simulink model "D_FB_J_controlled"  (R2020b)
(part 4 of 4)

                                                                                                                                                                                                                                                                                                                                                                                                                                                                                                                                                                                                                                                                                                                                                                                                                                                                                                                                                                                                                                                                                                                                                                                                                                                                                                                                                                                                                                                                                                                                                                                                                                                                                                                                                                                                                                                                                                                                                                                                                                                                                                                                                                                                  0.5000*a3B*dalfa*ml3B*offB*sin(th1B + th2B + th3B) + 0.5000*a3B*dbeta*ml3B*offB*sin(th1B + th2B + th3B) + 0.5000*L*a3B*dalfa*ml3B*sin(beta + th1B + th2B + th3B) + 0.5000*a1B*a3B*dalfa*ml3B*sin(th2B + th3B) + 0.5000*a1B*a3B*dbeta*ml3B*sin(th2B + th3B) + 0.5000*a1B*a3B*dth1B*ml3B*sin(th2B + th3B) + 0.5000*a2B*dalfa*ml2B*offB*sin(th1B + th2B) + a2B*dalfa*ml3B*offB*sin(th1B + th2B) + 0.5000*a2B*dbeta*ml2B*offB*sin(th1B + th2B) + a2B*dbeta*ml3B*offB*sin(th1B + th2B) + 0.5000*a1B*a2B*dalfa*ml2B*sin(th2B) + a1B*a2B*dalfa*ml3B*sin(th2B) + 0.5000*a1B*a2B*dbeta*ml2B*sin(th2B) + a1B*a2B*dbeta*ml3B*sin(th2B) + 0.5000*a1B*a2B*dth1B*ml2B*sin(th2B) + a1B*a2B*dth1B*ml3B*sin(th2B) - 0.5000*a2B*a3B*dth3B*ml3B*sin(th3B) + 0.5000*L*a2B*dalfa*ml2B*sin(beta + th1B + th2B) + L*a2B*dalfa*ml3B*sin(beta + th1B + th2B),                                                                                                                                                                                                                                                                                                                                                                                                                                                                                                                                                                                                                                                                                                                                                                                                                                                                                                                                                                                                                                                                                                                                                                                                                                                                                                                                                                                                                                                                                                                                                                                                                                                                                                                                                                                                                                                                                                                                                                                                                                                                                                                                                                                                                                                                                                                                                                                                                                                                                                                                                                                                                                                                                                                                                                                                                                                                                                                                                                                                                                                                                         0.5000*a3B*dalfa*ml3B*offB*sin(th1B + th2B + th3B) + 0.5000*a3B*dbeta*ml3B*offB*sin(th1B + th2B + th3B) + 0.5000*a1B*a3B*dalfa*ml3B*sin(th2B + th3B) + 0.5000*a1B*a3B*dbeta*ml3B*sin(th2B + th3B) + 0.5000*a1B*a3B*dth1B*ml3B*sin(th2B + th3B) + 0.5000*a2B*dalfa*ml2B*offB*sin(th1B + th2B) + a2B*dalfa*ml3B*offB*sin(th1B + th2B) + 0.5000*a2B*dbeta*ml2B*offB*sin(th1B + th2B) + a2B*dbeta*ml3B*offB*sin(th1B + th2B) + 0.5000*a1B*a2B*dalfa*ml2B*sin(th2B) + a1B*a2B*dalfa*ml3B*sin(th2B) + 0.5000*a1B*a2B*dbeta*ml2B*sin(th2B) + a1B*a2B*dbeta*ml3B*sin(th2B) + 0.5000*a1B*a2B*dth1B*ml2B*sin(th2B) + a1B*a2B*dth1B*ml3B*sin(th2B) - 0.5000*a2B*a3B*dth3B*ml3B*sin(th3B),                                                                                                                                                                                                                                                                                                                                                                                                                                                                                                                                                                                                                                                                                                                                                                                                                                                                                                                                                                                                                                                                                                                                                                                                                                                                                                                                                                                                                                                                                                                                                                                                                                                                                                                                                                                                                                                                                                                                                                                                                                                                                                                                                                                                0,                                                                                                                                                                                                                                                                                                                                                                                                                                                                                                                                                                                                                                                                                                                                                                                                                                                                                                                                                                                                                                                                                                                                                                                                                                                                                                                                                                                                                                                                                                                                                                                                                                                                                                                                                                                                                                                                        0,                                                                                                                                                                 0,                                                                                                                                                                                                                                                                                                                                                                                                                                                                                                                                                                                                                                                                                                                                                                                                                                                                                                                                                                                                                                                                                                                                                                                                                                                                                                                                                                                                                                                                                                                                                                                                                                                                                                                                                                                                                                                                             0.5000*a1B*dalfa*(a2B*ml2B*sin(th2B) + 2*a2B*ml3B*sin(th2B) + a3B*ml3B*sin(th2B + th3B)) + 0.5000*a1B*dbeta*(a2B*ml2B*sin(th2B) + 2*a2B*ml3B*sin(th2B) + a3B*ml3B*sin(th2B + th3B)) + 0.5000*a1B*dth1B*(a2B*ml2B*sin(th2B) + 2*a2B*ml3B*sin(th2B) + a3B*ml3B*sin(th2B + th3B)) - 0.5000*a2B*a3B*dth3B*ml3B*sin(th3B),                                                                                                                                                                                                                                                                                                                                                                                                                                                                                                                                                                                                                                                                                                                                                                                                                                                                                                                                                                                                                                                                                                                                                                                                                                                                                                                                                                                                                                                                                                                                                                                                                                                                                                                                                                                                                                     -0.5000*a2B*a3B*dth3B*ml3B*sin(th3B),                                                                                            -0.5000*a2B*a3B*ml3B*sin(th3B)*(dalfa + dbeta + dth1B + dth2B + dth3B); ...
                                                                                                                                                                                                                                                                                                                                                                                                                                                                                                                                                                                                                                                                                                                                                                                                                                                                                                                                                                                                                                                                                                                                                                                                                                                                                                                                                                                                                                                                                                                                                                                                                                                                                                                                                                                                                                                                                                                                                                                                                                                                                                                                                                                                                                                                                                                                                                                                                                                                                                                                                                                                                                                                                                                    0.5000*a3B*ml3B*(a2B*dalfa*sin(th3B) + a2B*dbeta*sin(th3B) + a2B*dth1B*sin(th3B) + a2B*dth2B*sin(th3B) + dalfa*offB*sin(th1B + th2B + th3B) + dbeta*offB*sin(th1B + th2B + th3B) + L*dalfa*sin(beta + th1B + th2B + th3B) + a1B*dalfa*sin(th2B + th3B) + a1B*dbeta*sin(th2B + th3B) + a1B*dth1B*sin(th2B + th3B)),                                                                                                                                                                                                                                                                                                                                                                                                                                                                                                                                                                                                                                                                                                                                                                                                                                                                                                                                                                                                                                                                                                                                                                                                                                                                                                                                                                                                                                                                                                                                                                                                                                                                                                                                                                                                                                                                                                                                                                                                                                                                                                                                                                                                                                                                                                                                                                                                                                                                                                                                                                                                                                                                                                                                                                                                                                                                                                                                                                                                                                                                                                                                                                                                                                                                                                                                                                                                                                                                                              0.5000*a3B*ml3B*(a2B*dalfa*sin(th3B) + a2B*dbeta*sin(th3B) + a2B*dth1B*sin(th3B) + a2B*dth2B*sin(th3B) + dalfa*offB*sin(th1B + th2B + th3B) + dbeta*offB*sin(th1B + th2B + th3B) + a1B*dalfa*sin(th2B + th3B) + a1B*dbeta*sin(th2B + th3B) + a1B*dth1B*sin(th2B + th3B)),                                                                                                                                                                                                                                                                                                                                                                                                                                                                                                                                                                                                                                                                                                                                                                                                                                                                                                                                                                                                                                                                                                                                                                                                                                                                                                                                                                                                                                                                                                                                                                                                                                                                                                                                                                                                                                                                                                                                                                                                                                                                                                                                                                                                0,                                                                                                                                                                                                                                                                                                                                                                                                                                                                                                                                                                                                                                                                                                                                                                                                                                                                                                                                                                                                                                                                                                                                                                                                                                                                                                                                                                                                                                                                                                                                                                                                                                                                                                                                                                                                                                                                        0,                                                                                                                                                                 0,                                                                                                                                                                                                                                                                                                                                                                                                                                                                                                                                                                                                                                                                                                                                                                                                                                                                                                                                                                                                                                                                                                                                                                                                                                                                                                                                                                                                                                                                                                                                                                                                                                                                                                                                                                                                                                                                                                                                                                                                   0.5000*a3B*ml3B*(a2B*dalfa*sin(th3B) + a2B*dbeta*sin(th3B) + a2B*dth1B*sin(th3B) + a2B*dth2B*sin(th3B) + a1B*dalfa*sin(th2B + th3B) + a1B*dbeta*sin(th2B + th3B) + a1B*dth1B*sin(th2B + th3B)),                                                                                                                                                                                                                                                                                                                                                                                                                                                                                                                                                                                                                                                                                                                                                                                                                                                                                                                                                                                                                                                                                                                                                                                                                                                                                                                                                                                                                                                                                                                                                                                                                                                                                                                                                                                                            0.5000*a2B*a3B*ml3B*sin(th3B)*(dalfa + dbeta + dth1B + dth2B),                                                                                                                                                                 0];
 
% Matrice Fv
Fv = diag([fv1p fv2p fv1A fv2A fv3A fv1B fv2B fv3B]);
  
% Vettore g
g = [- 0.5000*a2A*g0*ml2A*cos(alfa + beta + th1A + th2A) - a2A*g0*ml3A*cos(alfa + beta + th1A + th2A) - 0.5000*a2B*g0*ml2B*cos(alfa + beta + th1B + th2B) - a2B*g0*ml3B*cos(alfa + beta + th1B + th2B) - g0*ml1A*offA*cos(alfa + beta) - g0*ml2A*offA*cos(alfa + beta) - g0*ml1B*offB*cos(alfa + beta) - g0*ml3A*offA*cos(alfa + beta) - g0*ml2B*offB*cos(alfa + beta) - g0*ml3B*offB*cos(alfa + beta) - L*g0*m_base*cos(alfa) - 0.5000*L*g0*m_cavo*cos(alfa) - L*g0*ml1A*cos(alfa) - L*g0*ml1B*cos(alfa) - L*g0*ml2A*cos(alfa) - L*g0*ml2B*cos(alfa) - L*g0*ml3A*cos(alfa) - L*g0*ml3B*cos(alfa) - 0.5000*a3A*g0*ml3A*cos(alfa + beta + th1A + th2A + th3A) - 0.5000*a3B*g0*ml3B*cos(alfa + beta + th1B + th2B + th3B) - 0.5000*a1A*g0*ml1A*cos(alfa + beta + th1A) - a1A*g0*ml2A*cos(alfa + beta + th1A) - a1A*g0*ml3A*cos(alfa + beta + th1A) - 0.5000*a1B*g0*ml1B*cos(alfa + beta + th1B) - a1B*g0*ml2B*cos(alfa + beta + th1B) - a1B*g0*ml3B*cos(alfa + beta + th1B);
     - g0*ml2A*(0.5000*a2A*cos(alfa + beta + th1A + th2A) + offA*cos(alfa + beta) + a1A*cos(alfa + beta + th1A)) - g0*ml2B*(0.5000*a2B*cos(alfa + beta + th1B + th2B) + offB*cos(alfa + beta) + a1B*cos(alfa + beta + th1B)) - g0*ml3A*(a2A*cos(alfa + beta + th1A + th2A) + offA*cos(alfa + beta) + 0.5000*a3A*cos(alfa + beta + th1A + th2A + th3A) + a1A*cos(alfa + beta + th1A)) - g0*ml3B*(a2B*cos(alfa + beta + th1B + th2B) + offB*cos(alfa + beta) + 0.5000*a3B*cos(alfa + beta + th1B + th2B + th3B) + a1B*cos(alfa + beta + th1B)) - g0*ml1A*(offA*cos(alfa + beta) + 0.5000*a1A*cos(alfa + beta + th1A)) - g0*ml1B*(offB*cos(alfa + beta) + 0.5000*a1B*cos(alfa + beta + th1B));
     - g0*ml3A*(a2A*cos(alfa + beta + th1A + th2A) + 0.5000*a3A*cos(alfa + beta + th1A + th2A + th3A) + a1A*cos(alfa + beta + th1A)) - g0*ml2A*(0.5000*a2A*cos(alfa + beta + th1A + th2A) + a1A*cos(alfa + beta + th1A)) - 0.5000*a1A*g0*ml1A*cos(alfa + beta + th1A);
     - g0*ml3A*(a2A*cos(alfa + beta + th1A + th2A) + 0.5000*a3A*cos(alfa + beta + th1A + th2A + th3A)) - 0.5000*a2A*g0*ml2A*cos(alfa + beta + th1A + th2A);
     -0.5000*a3A*g0*ml3A*cos(alfa + beta + th1A + th2A + th3A);
     - g0*ml3B*(a2B*cos(alfa + beta + th1B + th2B) + 0.5000*a3B*cos(alfa + beta + th1B + th2B + th3B) + a1B*cos(alfa + beta + th1B)) - g0*ml2B*(0.5000*a2B*cos(alfa + beta + th1B + th2B) + a1B*cos(alfa + beta + th1B)) - 0.5000*a1B*g0*ml1B*cos(alfa + beta + th1B);
     - g0*ml3B*(a2B*cos(alfa + beta + th1B + th2B) + 0.5000*a3B*cos(alfa + beta + th1B + th2B + th3B)) - 0.5000*a2B*g0*ml2B*cos(alfa + beta + th1B + th2B);
     -0.5000*a3B*g0*ml3B*cos(alfa + beta + th1B + th2B + th3B)];

n = C*qd + Fv*qd + g;

% Scomposizione base - manipolatore 1 - manipolatore 2
Bb  = B(1:2,1:2);
Bb1 = B(1:2,3:5);
Bb2 = B(1:2,6:8);
B1b = B(3:5,1:2);
B1  = B(3:5,3:5);
B12 = B(3:5,6:8);
B2b = B(6:8,1:2);
B21 = B(6:8,3:5);
B2  = B(6:8,6:8);

nb = n(1:2);
n1 = n(3:5);
n2 = n(6:8);

% Partial FBL 
Bbm = B(1:2,3:8);
Bmb = B(3:8,1:2);
Bm  = B(3:8,3:8);
nm  = n(3:8);

B_tilde = Bm - Bmb*inv(Bb)*Bbm;
n_tilde = nm - Bmb*inv(Bb)*nb;

y1 = q0_ddot(1:3);
P_b2 = eye(3)-pinv(Bb2)*Bb2;
% y2 = pinv(Bb2)*(-Bb*qdd_pas-Bb1*y1-nb);
y2 = pinv(Bb2)*(-Bb*qdd_pas-Bb1*y1-nb) + P_b2*q0_ddot(4:6);
y = [y1; y2];
tau = B_tilde*y + n_tilde;

s_min = min(svd(Bb2));
r = rank(Bb2);

end
